simulink library "heli_2d_lib"  (Simulink 6.1)
values from neighbouring files (symbols this model uses):
  g = 9.81    [setup_heli_2d_configuration.m]
  J_eq_p = J_m_p + J_body_p + J_p + J_y    (= 0.0384309870395)    [setup_heli_2d_configuration.m]
  J_eq_y = J_m_y + J_body_y + J_p + J_y + J_shaft    (= 0.0431517259335)    [setup_heli_2d_configuration.m]
  K_CABLE_P = 5    [setup_lab_heli_2d.m]
  K_CABLE_Y = 3    [setup_lab_heli_2d.m]
  K_EC_P = - 2 * pi / ( 4 * 1024 )    (= -0.00153398078789)    [setup_lab_heli_2d.m]
  K_EC_Y = 2 * pi / ( 8 * 1024 )    (= 0.000766990393943)    [setup_lab_heli_2d.m]
  K_pp = K_f_p * r_p    (= 0.20413345)    [setup_heli_2d_configuration.m]
  K_py = K_t_y / R_m_y    (= 0.0068125)    [setup_heli_2d_configuration.m]
  K_yp = K_t_p / R_m_p    (= 0.0219277108434)    [setup_heli_2d_configuration.m]
  K_yy = K_f_y * r_y    (= 0.071988045)    [setup_heli_2d_configuration.m]
  l_cm = ( (m_motor_p + m_shield ) * r_p +  (m_motor_y + m_shield ) * r_y ) / ( m_props )    (= 0.185670125995)    [setup_heli_2d_configuration.m]
  m_heli = 1.3872    [setup_heli_2d_configuration.m]
  SAT_INT_ERR_PITCH = 5    [setup_lab_heli_2d.m]
  SAT_INT_ERR_YAW = 5    [setup_lab_heli_2d.m]
  theta_0 = 0    [setup_lab_heli_2d.m]
  Tr_p = 1    [setup_lab_heli_2d.m]
  Tr_y = 1    [setup_lab_heli_2d.m]
  VMAX_DAC = 10    [setup_lab_heli_2d.m]
  VMAX_UPM_P = 24    [setup_lab_heli_2d.m]
  VMAX_UPM_Y = 15    [setup_lab_heli_2d.m]
  wcf = 2 * pi * 20    (= 125.663706144)    [setup_lab_heli_2d.m]
  zetaf = 0.85    [setup_lab_heli_2d.m]
undefined symbols (not defined in the file or in its folder): B_p, B_y, K, Ki
libraries: qctools x4, simulink_extras x3, heli_2d_lib x2
settings Model: LastModifiedBy=MLevis  ExtModeArmWhenConnect=off

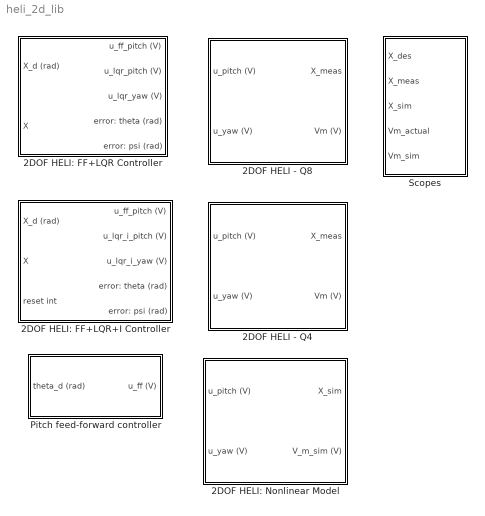
== system heli_2d_lib ==
  2DOF HELI - Q4 : Subsystem
  2DOF HELI - Q8 : Subsystem
  2DOF HELI: FF+LQR Controller : Subsystem
  2DOF HELI: FF+LQR+I Controller : Subsystem  AncestorBlock=heli_2d_lib/2DOF HELI: FF+LQR Controller
  2DOF HELI: Nonlinear Model : Subsystem  AncestorBlock=heli_2d_lib/2DOF Helicopter: Simple Nonlinear Model
  Pitch feed-forward controller : Subsystem  AncestorBlock=heli_2d_lib/2DOF HELI: FF+LQR+I Controller/Pitch feed-forward controller
  Scopes : Subsystem

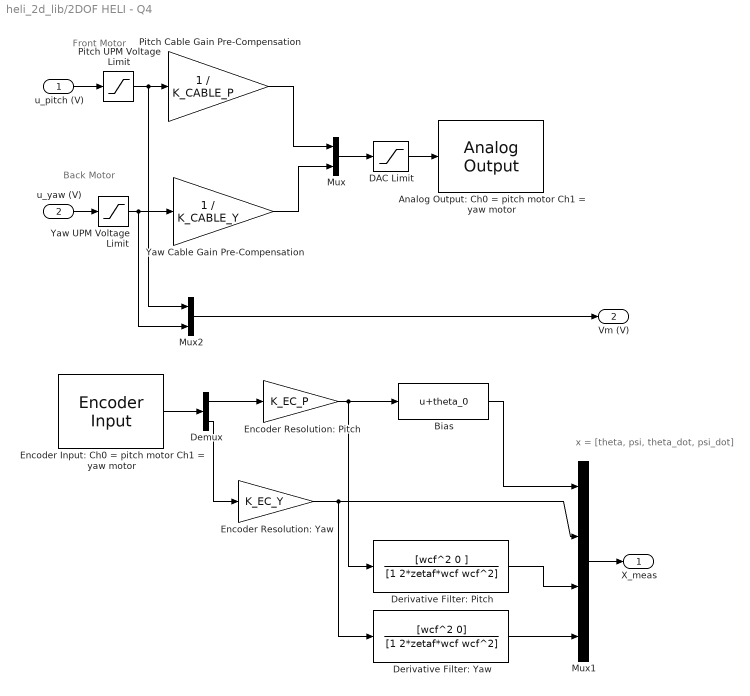
== system heli_2d_lib/2DOF HELI - Q4 ==
  note: Back Motor
  note: Front Motor
  note: x = [theta, psi, theta_dot, psi_dot]
  u_pitch (V) : Inport  Port=1  LatchInput=off
  u_yaw (V) : Inport  Port=2  LatchInput=off
  Analog Output: Ch0 = pitch motor Ch1 = yaw motor : qctools/Quanser Q4 Series/Analog Output  boardNumber=0  channels=[0,1]  modesVect=0  rangesVect=10  initialVect=0  finalVect=0  sampleTime=-1  inputVolts=on  simulationOutput=off
  Bias : Bias  Bias=theta_0
  DAC Limit : Saturate  UpperLimit=VMAX_DAC  LowerLimit=- VMAX_DAC
  Demux : Demux  Outputs=2
  Derivative Filter: Pitch : TransferFcn  Numerator=[wcf^2 0 ]  Denominator=[1 2*zetaf*wcf wcf^2]
  Derivative Filter: Yaw : TransferFcn  Numerator=[wcf^2 0]  Denominator=[1 2*zetaf*wcf wcf^2]
  Encoder Input: Ch0 = pitch motor Ch1 = yaw motor : qctools/Quanser Q4 Series/Encoder Input  boardNumber=0  channels=[0,1]  initial=0  preserveCounts=off  sampleTime=default_sample_time  quadratureStr=4X  modeStr=Normal  flagString=FLG1 is IDX and FLG2 is E  prescale=1  frequency=16666666.6667  use33MHzClock=off  bcd=off  enableIndex=on  synchronousIndex=on  indexPolarity=on  reloadOnIndex=off  simulationInput=off
  "Encoder Resolution: Pitch " : Gain  Gain=K_EC_P
  Encoder Resolution: Yaw : Gain  Gain=K_EC_Y
  Mux : Mux  Inputs=2
  Mux1 : Mux
  Mux2 : Mux  Inputs=2
  Pitch Cable Gain Pre-Compensation : Gain  Gain=1 / K_CABLE_P  SaturateOnIntegerOverflow=on
  Pitch UPM Voltage Limit : Saturate  UpperLimit=VMAX_UPM_P  LowerLimit=- VMAX_UPM_P
  Yaw Cable Gain Pre-Compensation : Gain  Gain=1 / K_CABLE_Y  SaturateOnIntegerOverflow=on
  Yaw UPM Voltage Limit : Saturate  UpperLimit=VMAX_UPM_Y  LowerLimit=- VMAX_UPM_Y
  X_meas : Outport
  Vm (V) : Outport  Port=2
  wires:
  Encoder Resolution: Yaw/1 -> Derivative Filter: Yaw/1, Mux1/2
  Mux2/1 -> Vm (V)/1
  Yaw Cable Gain Pre-Compensation/1 -> Mux/2
  Pitch Cable Gain Pre-Compensation/1 -> Mux/1
  Mux1/1 -> X_meas/1
  u_yaw (V)/1 -> Yaw UPM Voltage Limit/1
  u_pitch (V)/1 -> Pitch UPM Voltage Limit/1
  Yaw UPM Voltage Limit/1 -> Yaw Cable Gain Pre-Compensation/1, Mux2/2
  Pitch UPM Voltage Limit/1 -> Pitch Cable Gain Pre-Compensation/1, Mux2/1
  DAC Limit/1 -> Analog Output: Ch0 = pitch motor Ch1 = yaw motor/1
  Mux/1 -> DAC Limit/1
  Demux/1 -> "Encoder Resolution: Pitch "/1
  "Encoder Resolution: Pitch "/1 -> Derivative Filter: Pitch/1, Bias/1
  Encoder Input: Ch0 = pitch motor Ch1 = yaw motor/1 -> Demux/1
  Demux/2 -> Encoder Resolution: Yaw/1
  Bias/1 -> Mux1/1
  Derivative Filter: Pitch/1 -> Mux1/3
  Derivative Filter: Yaw/1 -> Mux1/4

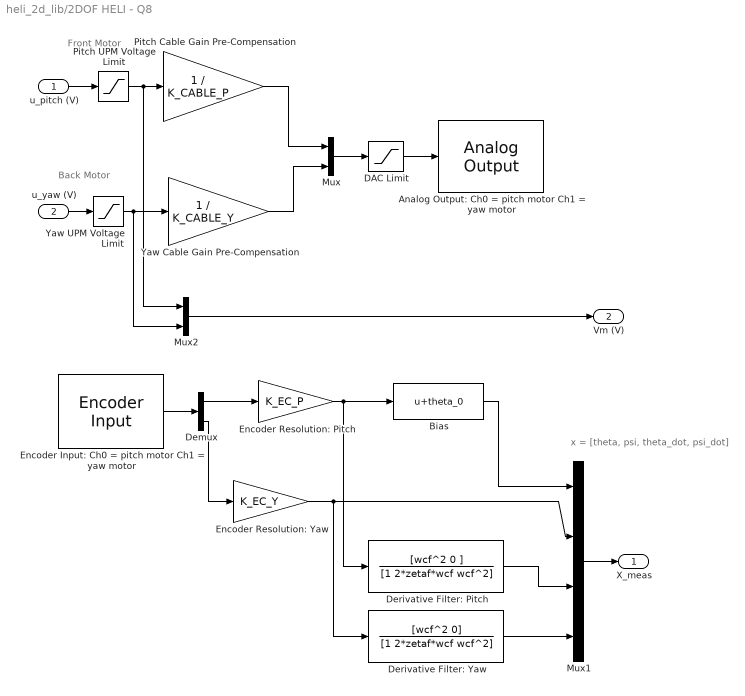
== system heli_2d_lib/2DOF HELI - Q8 ==
  note: x = [theta, psi, theta_dot, psi_dot]
  note: Front Motor
  note: Back Motor
  u_pitch (V) : Inport  Port=1  LatchInput=off
  u_yaw (V) : Inport  Port=2  LatchInput=off
  Analog Output: Ch0 = pitch motor Ch1 = yaw motor : qctools/Quanser Consulting Q8 Series/Analog Output  boardNumber=0  channels=[0,1]  modesVect=0  rangesVect=10  initialVect=0  finalVect=0  sampleTime=-1  inputVolts=on  simulationOutput=off
  Bias : Bias  Bias=theta_0
  DAC Limit : Saturate  UpperLimit=VMAX_DAC  LowerLimit=- VMAX_DAC
  Demux : Demux  Outputs=2
  Derivative Filter: Pitch : TransferFcn  Numerator=[wcf^2 0 ]  Denominator=[1 2*zetaf*wcf wcf^2]
  Derivative Filter: Yaw : TransferFcn  Numerator=[wcf^2 0]  Denominator=[1 2*zetaf*wcf wcf^2]
  Encoder Input: Ch0 = pitch motor Ch1 = yaw motor : qctools/Quanser Consulting Q8 Series/Encoder Input  boardNumber=0  channels=[0,1]  initial=0  preserveCounts=off  sampleTime=default_sample_time  quadratureStr=4X  modeStr=Normal  flagString=FLG1 is IDX and FLG2 is E  prescale=1  frequency=16666666.6667  bcd=off  enableIndex=on  synchronousIndex=on  indexPolarity=on  reloadOnIndex=off  simulationInput=off
  "Encoder Resolution: Pitch " : Gain  Gain=K_EC_P
  Encoder Resolution: Yaw : Gain  Gain=K_EC_Y
  Mux : Mux  Inputs=2
  Mux1 : Mux
  Mux2 : Mux  Inputs=2
  Pitch Cable Gain Pre-Compensation : Gain  Gain=1 / K_CABLE_P  SaturateOnIntegerOverflow=on
  Pitch UPM Voltage Limit : Saturate  UpperLimit=VMAX_UPM_P  LowerLimit=- VMAX_UPM_P
  Yaw Cable Gain Pre-Compensation : Gain  Gain=1 / K_CABLE_Y  SaturateOnIntegerOverflow=on
  Yaw UPM Voltage Limit : Saturate  UpperLimit=VMAX_UPM_Y  LowerLimit=- VMAX_UPM_Y
  X_meas : Outport
  Vm (V) : Outport  Port=2
  wires:
  Derivative Filter: Yaw/1 -> Mux1/4
  Derivative Filter: Pitch/1 -> Mux1/3
  Bias/1 -> Mux1/1
  Demux/2 -> Encoder Resolution: Yaw/1
  Encoder Input: Ch0 = pitch motor Ch1 = yaw motor/1 -> Demux/1
  "Encoder Resolution: Pitch "/1 -> Derivative Filter: Pitch/1, Bias/1
  Demux/1 -> "Encoder Resolution: Pitch "/1
  Mux/1 -> DAC Limit/1
  DAC Limit/1 -> Analog Output: Ch0 = pitch motor Ch1 = yaw motor/1
  Pitch UPM Voltage Limit/1 -> Pitch Cable Gain Pre-Compensation/1, Mux2/1
  Yaw UPM Voltage Limit/1 -> Yaw Cable Gain Pre-Compensation/1, Mux2/2
  u_pitch (V)/1 -> Pitch UPM Voltage Limit/1
  u_yaw (V)/1 -> Yaw UPM Voltage Limit/1
  Mux1/1 -> X_meas/1
  Pitch Cable Gain Pre-Compensation/1 -> Mux/1
  Yaw Cable Gain Pre-Compensation/1 -> Mux/2
  Mux2/1 -> Vm (V)/1
  Encoder Resolution: Yaw/1 -> Derivative Filter: Yaw/1, Mux1/2

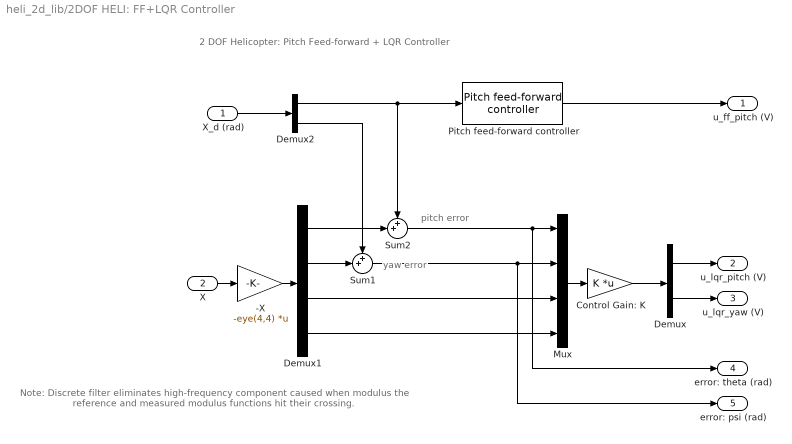
== system heli_2d_lib/2DOF HELI: FF+LQR Controller ==
  note: yaw error
  note: pitch error
  note: 2 DOF Helicopter:
      | Pitch Feed-forward + LQR Controller
  note: Note: Discrete filter eliminates high-frequency
      | component caused when modulus the reference
      | and measured modulus functions hit their crossing.
  X_d (rad) : Inport  Port=1  LatchInput=off
  X : Inport  Port=2  LatchInput=off
  -X : Gain  Gain=-eye(4,4)  Multiplication=Matrix(K*u)
  Control Gain: K : Gain  Gain=K  Multiplication=Matrix(K*u)
  Demux : Demux  Outputs=2
  Demux1 : Demux
  Demux2 : Demux  Outputs=2
  Mux : Mux
  Pitch feed-forward controller : heli_2d_lib/Pitch feed-forward controller
  Sum1 : Sum  Inputs=++|
  Sum2 : Sum  Inputs=++|
  u_ff_pitch (V) : Outport
  u_lqr_pitch (V) : Outport  Port=2
  u_lqr_yaw (V) : Outport  Port=3
  error: theta (rad) : Outport  Port=4
  error: psi (rad) : Outport  Port=5
  wires:
  Pitch feed-forward controller/1 -> u_ff_pitch (V)/1
  Demux/1 -> u_lqr_pitch (V)/1
  Demux/2 -> u_lqr_yaw (V)/1
  Sum2/1 -> Mux/1, error: theta (rad)/1
  Demux1/1 -> Sum2/2
  X/1 -> -X/1
  -X/1 -> Demux1/1
  Control Gain: K/1 -> Demux/1
  Mux/1 -> Control Gain: K/1
  Demux1/3 -> Mux/3
  Demux1/4 -> Mux/4
  X_d (rad)/1 -> Demux2/1
  Demux1/2 -> Sum1/2
  Demux2/2 -> Sum1/1
  Demux2/1 -> Pitch feed-forward controller/1, Sum2/1
  Sum1/1 -> Mux/2, error: psi (rad)/1

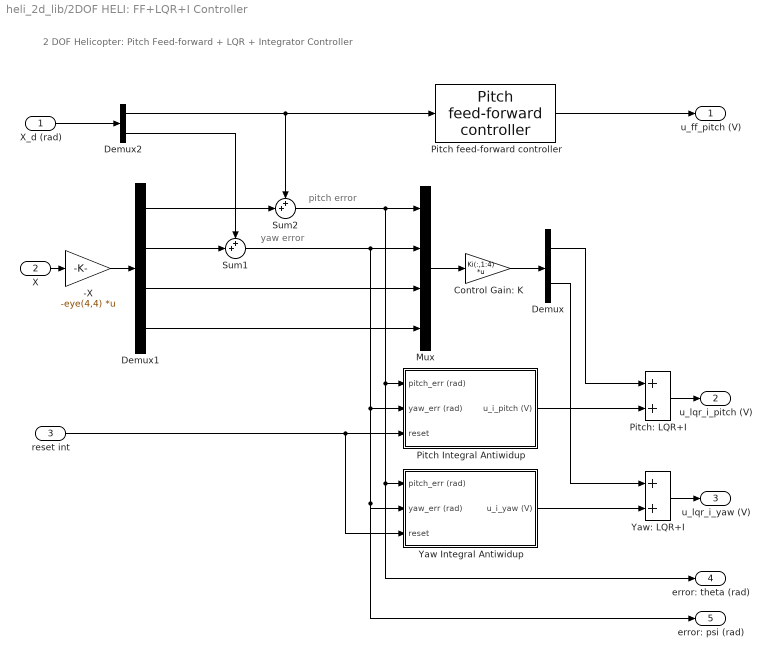
== system heli_2d_lib/2DOF HELI: FF+LQR+I Controller ==
  note: 2 DOF Helicopter:
      | Pitch Feed-forward + LQR + Integrator Controller
  note: pitch error
  note: yaw error
  X_d (rad) : Inport  Port=1  LatchInput=off
  X : Inport  Port=2  LatchInput=off
  reset int : Inport  Port=3  LatchInput=off
  -X : Gain  Gain=-eye(4,4)  Multiplication=Matrix(K*u)
  Control Gain: K : Gain  Gain=Ki(:,1:4)  Multiplication=Matrix(K*u)
  Demux : Demux  Outputs=2
  Demux1 : Demux
  Demux2 : Demux  Outputs=2
  Mux : Mux
  Pitch Integral Antiwidup : Subsystem  AncestorBlock=heli_2d_lib/2DOF HELI: FF+LQR+I Controller/Yaw Integral Antiwidup
  Pitch feed-forward controller : heli_2d_lib/Pitch feed-forward controller
  Pitch: LQR+I : Sum  OutScaling=2^-10
  Sum1 : Sum  Inputs=++|
  Sum2 : Sum  Inputs=++|
  Yaw Integral Antiwidup : Subsystem
  Yaw: LQR+I : Sum  OutScaling=2^-10
  u_ff_pitch (V) : Outport
  u_lqr_i_pitch (V) : Outport  Port=2
  u_lqr_i_yaw (V) : Outport  Port=3
  error: theta (rad) : Outport  Port=4
  error: psi (rad) : Outport  Port=5
  wires:
  Demux1/4 -> Mux/4
  Demux1/3 -> Mux/3
  Mux/1 -> Control Gain: K/1
  Control Gain: K/1 -> Demux/1
  -X/1 -> Demux1/1
  Sum1/1 -> Mux/2, Pitch Integral Antiwidup/2(yaw_err (rad)), error: psi (rad)/1, Yaw Integral Antiwidup/2(yaw_err (rad))
  X/1 -> -X/1
  Demux1/1 -> Sum2/2
  Sum2/1 -> Pitch Integral Antiwidup/1(pitch_err (rad)), error: theta (rad)/1, Yaw Integral Antiwidup/1(pitch_err (rad)), Mux/1
  Pitch feed-forward controller/1 -> u_ff_pitch (V)/1
  Pitch Integral Antiwidup/1(u_i_pitch (V)) -> Pitch: LQR+I/2
  Demux/1 -> Pitch: LQR+I/1
  Pitch: LQR+I/1 -> u_lqr_i_pitch (V)/1
  Yaw: LQR+I/1 -> u_lqr_i_yaw (V)/1
  Demux/2 -> Yaw: LQR+I/1
  Yaw Integral Antiwidup/1(u_i_yaw (V)) -> Yaw: LQR+I/2
  X_d (rad)/1 -> Demux2/1
  Demux2/1 -> Pitch feed-forward controller/1, Sum2/1
  Demux2/2 -> Sum1/1
  Demux1/2 -> Sum1/2
  reset int/1 -> Yaw Integral Antiwidup/3(reset), Pitch Integral Antiwidup/3(reset)

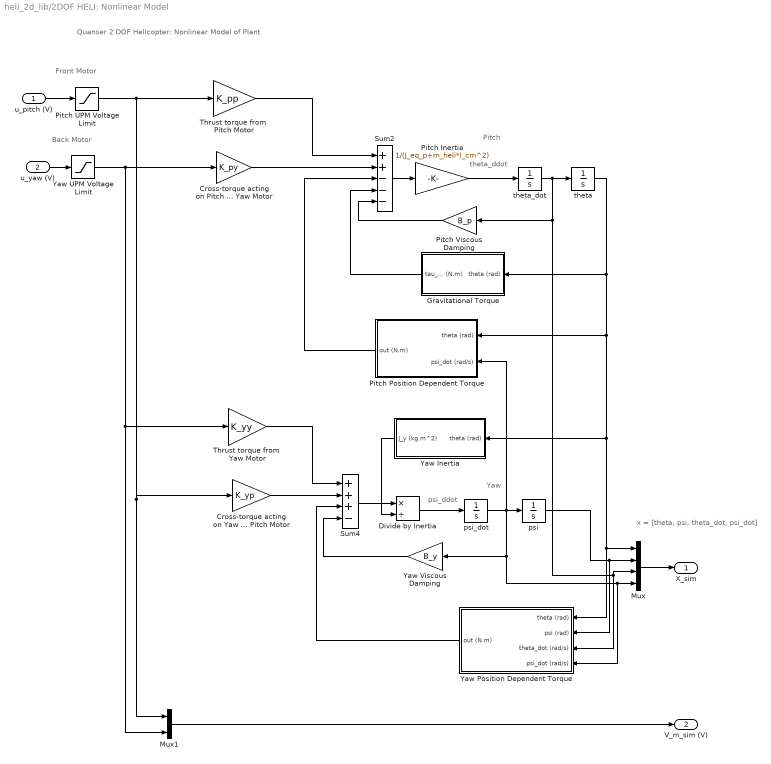
== system heli_2d_lib/2DOF HELI: Nonlinear Model ==
  note: Yaw
  note: Pitch
  note: psi_ddot
  note: theta_ddot
  note: Quanser 2 DOF Helicopter: Nonlinear Model of Plant
  note: x = [theta, psi, theta_dot, psi_dot]
  note: Front Motor
  note: Back Motor
  u_pitch (V) : Inport  Port=1  LatchInput=off
  u_yaw (V) : Inport  Port=2  LatchInput=off
  Cross-torque acting on Pitch  from Yaw Motor : Gain  Gain=K_py
  Cross-torque acting on Yaw  from Pitch Motor : Gain  Gain=K_yp
  Divide by Inertia : Product  Inputs=*/  OutScaling=2^-10
  Gravitational Torque : Subsystem  Orientation=left
  Mux : Mux
  Mux1 : Mux  Inputs=2
  Pitch Inertia : Gain  Gain=1/(J_eq_p+m_heli*l_cm^2)
  Pitch Position Dependent Torque : Subsystem  Orientation=left  AncestorBlock=heli_2d_lib/2DOF Helicopter: Nonlinear Model/Yaw Nonlinear Element
  Pitch UPM Voltage Limit : Saturate  UpperLimit=VMAX_UPM_P  LowerLimit=- VMAX_UPM_P
  Pitch Viscous Damping : Gain  Orientation=left  Gain=B_p
  Sum2 : Sum  Inputs=++---
  Sum4 : Sum  Inputs=+++-
  Thrust torque from  Pitch Motor : Gain  Gain=K_pp
  Thrust torque from  Yaw Motor : Gain  Gain=K_yy
  Yaw Inertia : Subsystem  Orientation=left
  Yaw Position Dependent Torque : Subsystem  Orientation=left
  Yaw UPM Voltage Limit : Saturate  UpperLimit=VMAX_UPM_Y  LowerLimit=- VMAX_UPM_Y
  Yaw Viscous Damping : Gain  Orientation=left  Gain=B_y
  psi : Integrator
  psi_dot : Integrator
  theta : Integrator  InitialCondition=theta_0  LimitOutput=on  UpperSaturationLimit=40.5*pi/180  LowerSaturationLimit=-40.5*pi/180
  theta_dot : Integrator
  X_sim : Outport
  V_m_sim (V) : Outport  Port=2
  wires:
  u_yaw (V)/1 -> Yaw UPM Voltage Limit/1
  u_pitch (V)/1 -> Pitch UPM Voltage Limit/1
  psi_dot/1 -> psi/1, Pitch Position Dependent Torque/2(psi_dot (rad/s)), Mux/4, Yaw Position Dependent Torque/4(psi_dot (rad/s)), Yaw Viscous Damping/1
  Cross-torque acting on Yaw  from Pitch Motor/1 -> Sum4/2
  Thrust torque from  Yaw Motor/1 -> Sum4/1
  theta_dot/1 -> theta/1, Mux/3, Yaw Position Dependent Torque/3(theta_dot (rad/s)), Pitch Viscous Damping/1
  Pitch Inertia/1 -> theta_dot/1
  Sum2/1 -> Pitch Inertia/1
  theta/1 -> Yaw Inertia/1(theta (rad)), Mux/1, Yaw Position Dependent Torque/1(theta (rad)), Pitch Position Dependent Torque/1(theta (rad)), Gravitational Torque/1(theta (rad))
  Mux/1 -> X_sim/1
  Pitch UPM Voltage Limit/1 -> Thrust torque from  Pitch Motor/1, Mux1/1, Cross-torque acting on Yaw  from Pitch Motor/1
  Yaw UPM Voltage Limit/1 -> Cross-torque acting on Pitch  from Yaw Motor/1, Mux1/2, Thrust torque from  Yaw Motor/1
  Mux1/1 -> V_m_sim (V)/1
  psi/1 -> Mux/2, Yaw Position Dependent Torque/2(psi (rad))
  Yaw Viscous Damping/1 -> Sum4/4
  Yaw Position Dependent Torque/1(out (N.m)) -> Sum4/3
  Sum4/1 -> Divide by Inertia/1
  Divide by Inertia/1 -> psi_dot/1
  Yaw Inertia/1(J_y (kg.m^2)) -> Divide by Inertia/2
  Thrust torque from  Pitch Motor/1 -> Sum2/1
  Cross-torque acting on Pitch  from Yaw Motor/1 -> Sum2/2
  Pitch Viscous Damping/1 -> Sum2/5
  Gravitational Torque/1(tau_g (N.m)) -> Sum2/4
  Pitch Position Dependent Torque/1(out (N.m)) -> Sum2/3

== system heli_2d_lib/Pitch feed-forward controller ==
  note: Desired pitch angle
  theta_d (rad) : Inport  Port=1  LatchInput=off
  Feed-forward Pitch Gain : Gain  Gain=l_cm*m_heli*g / K_pp
  Trigonometric Function : Trigonometry  Operator=cos  OutputSignalType=real
  u_ff (V) : Outport
  wires:
  Trigonometric Function/1 -> Feed-forward Pitch Gain/1
  Feed-forward Pitch Gain/1 -> u_ff (V)/1
  theta_d (rad)/1 -> Trigonometric Function/1

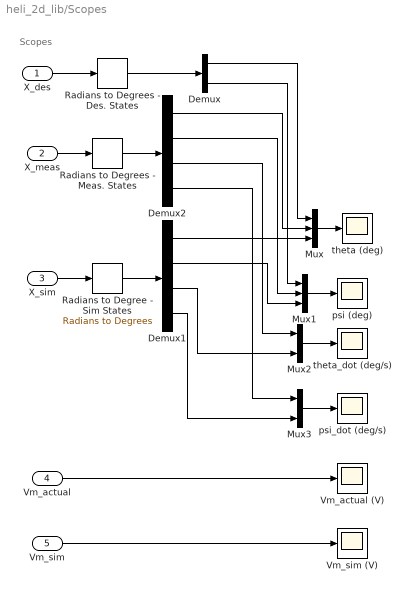
== system heli_2d_lib/Scopes ==
  note: Scopes
  X_des : Inport  Port=1  LatchInput=off
  X_meas : Inport  Port=2  LatchInput=off
  X_sim : Inport  Port=3  LatchInput=off
  Vm_actual : Inport  Port=4  LatchInput=off
  Vm_sim : Inport  Port=5  LatchInput=off
  Demux : Demux  Outputs=2
  Demux1 : Demux
  Demux2 : Demux
  Mux : Mux  Inputs=3
  Mux1 : Mux  Inputs=3
  Mux2 : Mux  Inputs=2
  Mux3 : Mux  Inputs=2
  Radians to Degree - Sim States : simulink_extras/Transformations/Radians to Degrees
  Radians to Degrees - Des. States : simulink_extras/Transformations/Radians to Degrees
  Radians to Degrees - Meas. States : simulink_extras/Transformations/Radians to Degrees
  Vm_actual (V) : Scope
      settings: TickLabels=on  TimeRange=1.000000  YMin=-250  YMax=250  SaveName=ScopeData4  DataFormat=Array
  Vm_sim (V) : Scope
      settings: TickLabels=on  TimeRange=1.000000  YMin=-250  YMax=250  SaveName=ScopeData5  DataFormat=Array
  psi (deg) : Scope
      settings: TickLabels=on  TimeRange=50  YMin=-5.5  YMax=5.5  DataFormat=Array
  psi_dot (deg/s) : Scope
      settings: TickLabels=on  TimeRange=1.000000  YMin=-250  YMax=250  SaveName=ScopeData3  DataFormat=Array
  theta (deg) : Scope
      settings: TickLabels=on  TimeRange=50  YMin=-15  YMax=15  DataFormat=Array
  theta_dot (deg/s) : Scope
      settings: TickLabels=on  TimeRange=1.000000  YMin=-250  YMax=250  SaveName=ScopeData2  DataFormat=Array
  wires:
  Vm_actual/1 -> Vm_actual (V)/1
  Demux1/4 -> Mux3/2
  Demux1/3 -> Mux2/2
  Mux3/1 -> psi_dot (deg/s)/1
  Mux2/1 -> theta_dot (deg/s)/1
  Mux1/1 -> psi (deg)/1
  Mux/1 -> theta (deg)/1
  Radians to Degree - Sim States/1 -> Demux1/1
  X_sim/1 -> Radians to Degree - Sim States/1
  Radians to Degrees - Meas. States/1 -> Demux2/1
  X_meas/1 -> Radians to Degrees - Meas. States/1
  Demux2/4 -> Mux3/1
  Demux2/3 -> Mux2/1
  X_des/1 -> Radians to Degrees - Des. States/1
  Demux/1 -> Mux/1
  Demux2/1 -> Mux/2
  Demux1/1 -> Mux/3
  Demux/2 -> Mux1/1
  Demux2/2 -> Mux1/2
  Demux1/2 -> Mux1/3
  Radians to Degrees - Des. States/1 -> Demux/1
  Vm_sim/1 -> Vm_sim (V)/1

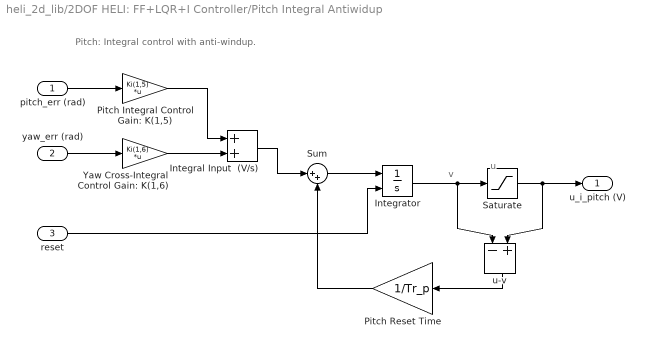
== system heli_2d_lib/2DOF HELI: FF+LQR+I Controller/Pitch Integral Antiwidup ==
  note: u
  note: v
  note: Pitch: Integral control with anti-windup.
  pitch_err (rad) : Inport  Port=1  LatchInput=off
  yaw_err (rad) : Inport  Port=2  LatchInput=off
  reset : Inport  Port=3  LatchInput=off
  Integral Input  (V/s) : Sum  OutScaling=2^-10
  Integrator : Integrator  ExternalReset=rising
  Pitch Integral Control Gain: K(1,5) : Gain  Gain=Ki(1,5)  Multiplication=Matrix(K*u)
  Pitch Reset Time : Gain  Orientation=left  Gain=1/Tr_p
  Saturate : Saturate  UpperLimit=SAT_INT_ERR_PITCH  LowerLimit=-SAT_INT_ERR_PITCH
  Sum : Sum  Inputs=|++
  Yaw Cross-Integral Control Gain: K(1,6) : Gain  Gain=Ki(1,6)  Multiplication=Matrix(K*u)
  u-v : Sum  Orientation=down  Inputs=-+  OutScaling=2^-10
  u_i_pitch (V) : Outport
  wires:
  pitch_err (rad)/1 -> Pitch Integral Control Gain: K(1,5)/1
  Integrator/1 -> u-v/1, Saturate/1
  Saturate/1 -> u_i_pitch (V)/1, u-v/2
  u-v/1 -> Pitch Reset Time/1
  Sum/1 -> Integrator/1
  Pitch Reset Time/1 -> Sum/2
  reset/1 -> Integrator/2
  yaw_err (rad)/1 -> Yaw Cross-Integral Control Gain: K(1,6)/1
  Pitch Integral Control Gain: K(1,5)/1 -> Integral Input  (V/s)/1
  Yaw Cross-Integral Control Gain: K(1,6)/1 -> Integral Input  (V/s)/2
  Integral Input  (V/s)/1 -> Sum/1

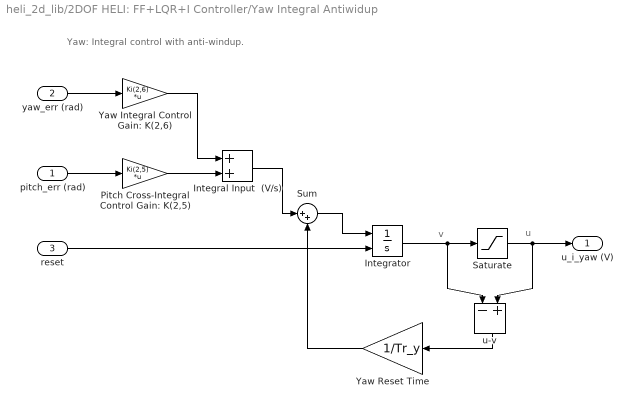
== system heli_2d_lib/2DOF HELI: FF+LQR+I Controller/Yaw Integral Antiwidup ==
  note: v
  note: u
  note: Yaw: Integral control with anti-windup.
  pitch_err (rad) : Inport  Port=1  LatchInput=off
  yaw_err (rad) : Inport  Port=2  LatchInput=off
  reset : Inport  Port=3  LatchInput=off
  Integral Input  (V/s) : Sum  OutScaling=2^-10
  Integrator : Integrator  ExternalReset=rising
  Pitch Cross-Integral Control Gain: K(2,5) : Gain  Gain=Ki(2,5)  Multiplication=Matrix(K*u)
  Saturate : Saturate  UpperLimit=SAT_INT_ERR_YAW  LowerLimit=-SAT_INT_ERR_YAW
  Sum : Sum  Inputs=|++
  Yaw Integral Control Gain: K(2,6) : Gain  Gain=Ki(2,6)  Multiplication=Matrix(K*u)
  Yaw Reset Time : Gain  Orientation=left  Gain=1/Tr_y
  u-v : Sum  Orientation=down  Inputs=-+  OutScaling=2^-10
  u_i_yaw (V) : Outport
  wires:
  Yaw Reset Time/1 -> Sum/2
  Sum/1 -> Integrator/1
  u-v/1 -> Yaw Reset Time/1
  Saturate/1 -> u-v/2, u_i_yaw (V)/1
  Integrator/1 -> Saturate/1, u-v/1
  yaw_err (rad)/1 -> Yaw Integral Control Gain: K(2,6)/1
  reset/1 -> Integrator/2
  pitch_err (rad)/1 -> Pitch Cross-Integral Control Gain: K(2,5)/1
  Yaw Integral Control Gain: K(2,6)/1 -> Integral Input  (V/s)/1
  Pitch Cross-Integral Control Gain: K(2,5)/1 -> Integral Input  (V/s)/2
  Integral Input  (V/s)/1 -> Sum/1

== system heli_2d_lib/2DOF HELI: Nonlinear Model/Gravitational Torque ==
  theta (rad) : Inport  Port=1  LatchInput=off
  Trigonometric Function : Trigonometry  Operator=cos  OutputSignalType=real
  m*g*lcm : Gain  Gain=m_heli*g*l_cm
  tau_g (N.m) : Outport
  wires:
  Trigonometric Function/1 -> m*g*lcm/1
  theta (rad)/1 -> Trigonometric Function/1
  m*g*lcm/1 -> tau_g (N.m)/1

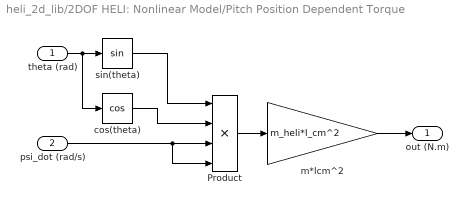
== system heli_2d_lib/2DOF HELI: Nonlinear Model/Pitch Position Dependent Torque ==
  theta (rad) : Inport  Port=1  LatchInput=off
  psi_dot (rad/s) : Inport  Port=2  LatchInput=off
  Product : Product  Inputs=4  RndMeth=Zero
  cos(theta) : Trigonometry  Operator=cos  OutputSignalType=real
  m*lcm^2 : Gain  Gain=m_heli*l_cm^2
  sin(theta) : Trigonometry  OutputSignalType=real
  out (N.m) : Outport
  wires:
  m*lcm^2/1 -> out (N.m)/1
  cos(theta)/1 -> Product/2
  sin(theta)/1 -> Product/1
  Product/1 -> m*lcm^2/1
  theta (rad)/1 -> sin(theta)/1, cos(theta)/1
  psi_dot (rad/s)/1 -> Product/3, Product/4

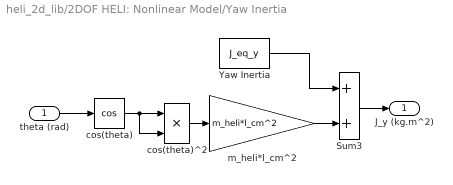
== system heli_2d_lib/2DOF HELI: Nonlinear Model/Yaw Inertia ==
  theta (rad) : Inport  Port=1  LatchInput=off
  Sum3 : Sum
  Yaw Inertia : Constant  Value=J_eq_y
  cos(theta) : Trigonometry  Operator=cos  OutputSignalType=real
  cos(theta)^2 : Product  RndMeth=Zero
  m_heli*l_cm^2 : Gain  Gain=m_heli*l_cm^2
  J_y (kg.m^2) : Outport
  wires:
  cos(theta)^2/1 -> m_heli*l_cm^2/1
  Yaw Inertia/1 -> Sum3/1
  m_heli*l_cm^2/1 -> Sum3/2
  theta (rad)/1 -> cos(theta)/1
  Sum3/1 -> J_y (kg.m^2)/1
  cos(theta)/1 -> cos(theta)^2/1, cos(theta)^2/2

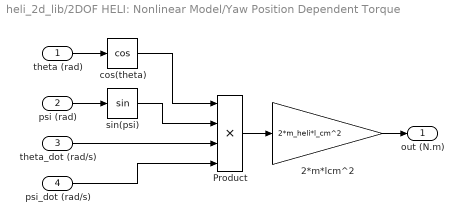
== system heli_2d_lib/2DOF HELI: Nonlinear Model/Yaw Position Dependent Torque ==
  theta (rad) : Inport  Port=1  LatchInput=off
  psi (rad) : Inport  Port=2  LatchInput=off
  theta_dot (rad/s) : Inport  Port=3  LatchInput=off
  psi_dot (rad/s) : Inport  Port=4  LatchInput=off
  2*m*lcm^2 : Gain  Gain=2*m_heli*l_cm^2
  Product : Product  Inputs=4  RndMeth=Zero
  cos(theta) : Trigonometry  Operator=cos  OutputSignalType=real
  sin(psi) : Trigonometry  OutputSignalType=real
  out (N.m) : Outport
  wires:
  psi (rad)/1 -> sin(psi)/1
  theta (rad)/1 -> cos(theta)/1
  Product/1 -> 2*m*lcm^2/1
  cos(theta)/1 -> Product/1
  sin(psi)/1 -> Product/2
  theta_dot (rad/s)/1 -> Product/3
  psi_dot (rad/s)/1 -> Product/4
  2*m*lcm^2/1 -> out (N.m)/1
